simulink model "hevmpcfixed"  (R2016b)
settings: Solver=FixedStepAuto  StartTime=0.0  StopTime=100  RelTol=1e-3
undefined symbols (not defined in the file or in its folder): F, G, k1, k2, k3, k4, N, P_req, Q0, Q1, Q2, Ts, ubounds, x0, zbounds
undefined symbols (not defined in the file): Mz
settings Model: Creator=Niklas  LastModifiedBy=Niklas
settings DataIOCC: SaveTime=off

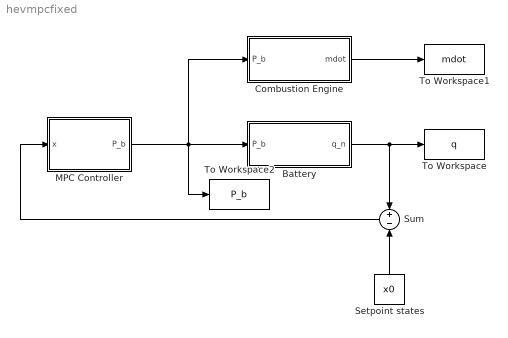
== system hevmpcfixed ==
  Battery : Subsystem  mask{k1=k1, k2=k2, k3=k3, k4=k4}
      mask DialogControl Control2 Prompt: Uoc = k2*q + k1
      mask DialogControl Control3 Prompt: R_i = k4*q + k3
  Combustion Engine : Subsystem  mask{c_f=0.0874}
  MPC Controller : Subsystem  mask{F=F, G=G, M=Mz, N=N, Q1=Q1, Q2=Q2, ubounds=ubounds, Ts=Ts, ufname='solvempcproblem', P_req=P_req, zbounds=zbounds}
      mask prompts: ubounds "Input bounds [u1min u1max;u2min u2max;...]"; ufname "Output function (Ex: 'myfun1')"
      mask Display:
      | port_label('input',1,'x')
      | port_label('output',1,'u')
  Setpoint states : Constant  Value=x0
  Sum : Sum  Inputs=+|-
  To Workspace : ToWorkspace  VariableName=q  SampleTime=-1
  To Workspace1 : ToWorkspace  VariableName=mdot  SampleTime=-1
  To Workspace2 : ToWorkspace  VariableName=P_b  SampleTime=-1
  wires:
  MPC Controller/1(P_b) -> To Workspace2/1, Battery/1(P_b), Combustion Engine/1(P_b)
  Battery/1(q_n) -> Sum/1, To Workspace/1
  Setpoint states/1 -> Sum/2
  Sum/1 -> MPC Controller/1(x)
  Combustion Engine/1(mdot) -> To Workspace1/1

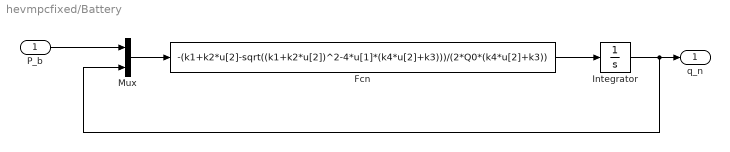
== system hevmpcfixed/Battery ==
  P_b : Inport
  Fcn : Fcn  Expr=-(k1+k2*u[2]-sqrt((k1+k2*u[2])^2-4*u[1]*(k4*u[2]+k3)))/(2*Q0*(k4*u[2]+k3))
  Integrator : Integrator  InitialCondition=x0(1)
  Mux : Mux  Inputs=2
  q_n : Outport
  wires:
  Fcn/1 -> Integrator/1
  Integrator/1 -> q_n/1, Mux/2
  P_b/1 -> Mux/1
  Mux/1 -> Fcn/1

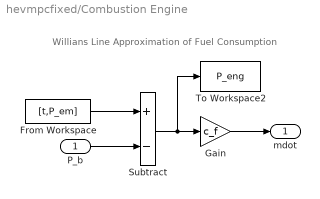
== system hevmpcfixed/Combustion Engine ==
  note: Willians Line Approximation of Fuel Consumption
  P_b : Inport
  From Workspace : FromWorkspace  VariableName=[t,P_em]  SampleTime=0
  Gain : Gain  Gain=c_f
  Subtract : Sum  Inputs=+-
  To Workspace2 : ToWorkspace  VariableName=P_eng  SampleTime=-1
  mdot : Outport
  wires:
  Gain/1 -> mdot/1
  Subtract/1 -> To Workspace2/1, Gain/1
  From Workspace/1 -> Subtract/1
  P_b/1 -> Subtract/2

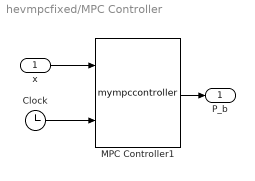
== system hevmpcfixed/MPC Controller ==
  x : Inport
  Clock : Clock
  MPC Controller1 : M-S-Function  FunctionName=mympccontroller  Parameters=F,G,M,N,Q1,Q2,ubounds,Ts,ufname,P_req,zbounds  mask{F=F, G=G, M=M, N=N, Q1=Q1, Q2=Q2, ubounds=ubounds, Ts=Ts, ufname=ufname, P_req=P_req, zbounds=zbounds}
      mask prompts: ubounds "ubounds [u1min u1max;u2min u2max;...]"; ufname "Output function (Ex: 'myfun1')"
      mask Display:
      | port_label('input',1,'x')
      | port_label('input',2,'t')
      | port_label('output',1,'u')
  P_b : Outport
  wires:
  MPC Controller1/1 -> P_b/1
  Clock/1 -> MPC Controller1/2
  x/1 -> MPC Controller1/1
